simulink model "sun_vec"  (R2024b)
settings: Solver=VariableStepAuto  StartTime=0.0  StopTime=326  RelTol=1e-3
values from neighbouring files (symbols this model uses):
  s_body_interp = cell(length(CV_folders), 1)    [SunVector_Characterize.m]
undefined symbols (not defined in the file or in its folder): ss_p_m
libraries: vrlib x2, aerolibutil x1, simulink x1
settings Model: Creator=zhasi  LastModifiedBy=zhasi

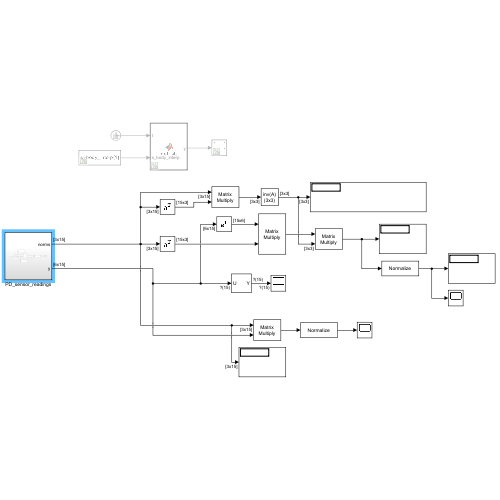
[thumbnail: Simulink's stored preview of the top-level diagram]
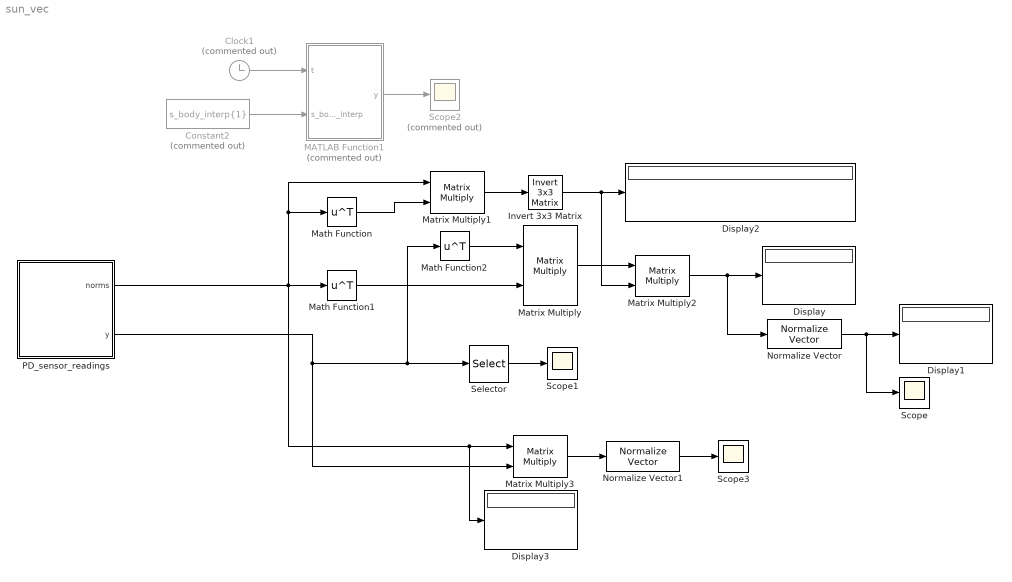
== system sun_vec ==
  Clock1 : Clock  Commented=on
  Constant2 : Constant  Commented=on  Value=s_body_interp{1}
  Display{,1..3} (4 alike) : Display
  Invert 3x3 Matrix : aerolibutil/Invert  3x3 Matrix
  MATLAB Function1 : MATLAB Function  Commented=on  TreatAsAtomicUnit=on
  Math Function : Math  Operator=transpose
  Math Function1 : Math  Operator=transpose
  Math Function2 : Math  Operator=transpose
  Matrix Multiply{,1..3} (4 alike) : Product  Multiplication=Matrix(*)
  Normalize Vector : vrlib/Utilities/Normalize Vector  maxzero=0
  Normalize Vector1 : vrlib/Utilities/Normalize Vector  maxzero=0
  PD_sensor_readings : Subsystem
  Scope : Scope
  Scope1 : Scope
  Scope2 : Scope  Commented=on
  Scope3 : Scope
  Selector : Selector  InputPortWidth=15  IndexOptions=Index vector (dialog)  Indices=[1:15]  OutputSizes=1
  wires:
  Clock1/1 -> MATLAB Function1/1(t)
  Math Function/1 -> Matrix Multiply1/2
  Constant2/1 -> MATLAB Function1/2(s_body_interp)
  MATLAB Function1/1(y) -> Scope2/1
  Math Function1/1 -> Matrix Multiply/2
  Invert 3x3 Matrix/1 -> Matrix Multiply2/2, Display2/1
  Matrix Multiply1/1 -> Invert 3x3 Matrix/1
  Matrix Multiply/1 -> Matrix Multiply2/1
  Math Function2/1 -> Matrix Multiply/1
  Matrix Multiply2/1 -> Normalize Vector/1, Display/1
  Normalize Vector/1 -> Scope/1, Display1/1
  Matrix Multiply3/1 -> Normalize Vector1/1
  Normalize Vector1/1 -> Scope3/1
  Selector/1 -> Scope1/1
  PD_sensor_readings/1(norms) -> Display3/1, Matrix Multiply3/1, Matrix Multiply1/1, Math Function/1, Math Function1/1
  PD_sensor_readings/2(y) -> Matrix Multiply3/2, Selector/1, Math Function2/1

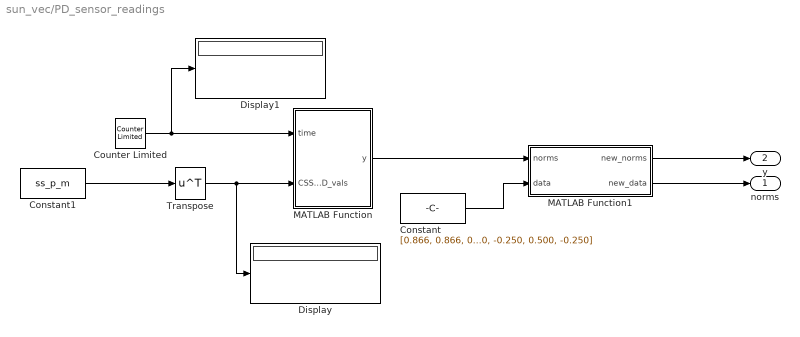
== system sun_vec/PD_sensor_readings ==
  Constant : Constant  Value=[0.866, 0.866, 0.866, 0.500, 0.500, 0.000, 0.500, 0.000, 0.000, 0.500, 0.000, 0.000, -0.866, -0.866, -0.866; 0.000, -0.433, 0.433, 0.866, -0.866, -0.866, 0.866, 0.866, 0.866, -0.866, -0.866, 0.000, -0.433, 0.000, 0.433; -0.500, 0.250, 0.250, 0.000, 0.000, -0.500, 0.000, -0.500, 0.500, 0.000, 0.500, 1.000, -0.250, 0.500, -0.250]
  Constant1 : Constant  Value=ss_p_m
  Counter Limited : simulink/Sources/Counter Limited  uplimit=327  tsamp=1
  Display : Display
  Display1 : Display
  MATLAB Function : MATLAB Function  TreatAsAtomicUnit=on
  MATLAB Function1 : MATLAB Function  TreatAsAtomicUnit=on
  Transpose : Math  Operator=transpose
  norms : Outport
  y : Outport  Port=2
  wires:
  Constant1/1 -> Transpose/1
  Transpose/1 -> MATLAB Function/2(CSS_AD_vals), Display/1
  Counter Limited/1 -> MATLAB Function/1(time), Display1/1
  MATLAB Function/1(y) -> MATLAB Function1/1(norms)
  MATLAB Function1/1(new_norms) -> y/1
  Constant/1 -> MATLAB Function1/2(data)
  MATLAB Function1/2(new_data) -> norms/1

== matlab function sun_vec/MATLAB Function1 ==
  data: t input; y output; s_body_interp input
function y = get_sb(t, s_body_interp)

idx = floor(t)+1;
% for i = 1:4
%     CSS_AD_vals(1,:) = CSS_AD_vals(1,:) - min(CSS_AD_vals(1,:));
% end
y = s_body_interp(:, idx);

== matlab function sun_vec/PD_sensor_readings/MATLAB Function ==
  data: time input; y output; CSS_AD_vals input
function y = get_b(time, CSS_AD_vals)

% means = zeros(5);
% % 1. Find the average value for each CSS board
% for i = 1:5 %iterate through CSS boards
%     means(i) = mean(CSS_AD_vals((4*i:(4*i+4))));
% end

idx = time+1;

% 2. Zero out all individual PDs that are below the voltage threshold
voltage_threshold = 2750;
% for i = 1:16
for i = 1:15
    if (CSS_AD_vals(i, idx) < voltage_threshold)
        % CSS_AD_vals(i, idx) = NaN;
        CSS_AD_vals(i, idx) = 0;
    end
end

% 3. Take values from remaining highest 3 CSS boards
% [~, sorted_indices] = sort(means(1:5), 'descend');
% invalid_boards = sorted_indices(4:5);

% CSS_AD_vals(1+4*invalid_boards(1):4+4*invalid_boards(1)) = [0; 0; 0; 0];
% CSS_AD_vals(1+4*invalid_boards(2):4+4*invalid_boards(2)) = [0; 0; 0; 0];

y = CSS_AD_vals(:, idx);

== matlab function sun_vec/PD_sensor_readings/MATLAB Function1 ==
  data: norms input; new_norms output; data input; new_data output
function [new_norms, new_data] = fcn(norms, data)
%#codegen
% [new_data, idx] = maxk(data, 6);
% new_norms = zeros(6, size(norms,1), 'like', norms);
% new_norms(:, :) = norms(idx);
% new_norms = new_norms';
    new_norms = norms;
    new_data = data;
end
